simulink model "scheme1_analysis"  (R2019b)
settings: Solver=ode4  StartTime=0.0  StopTime=30  FixedStep=0.1  RelTol=1e-3
values from neighbouring files (symbols this model uses):
  Kd = K(3)    [solution.m]
  Ki = K(1)    [solution.m]
  Kp = K(2)    [solution.m]
settings Model: Creator=biannic  LastModifiedBy=biannic
settings DataIOCC: ReturnWorkspaceOutputs=off

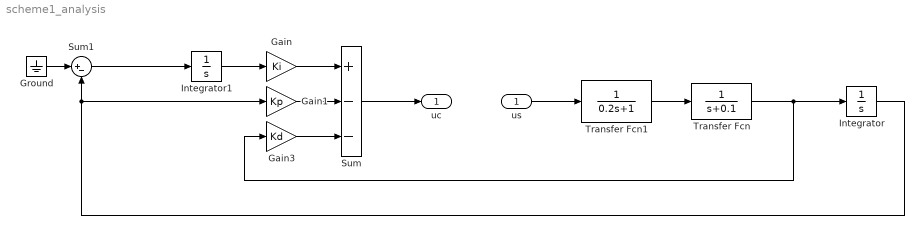
== system scheme1_analysis ==
  us : Inport
  Gain : Gain  Gain=Ki
  Gain1 : Gain  Gain=Kp
  Gain3 : Gain  Gain=Kd
  Ground : Ground
  Integrator : Integrator
  Integrator1 : Integrator
  Sum : Sum  Inputs=+--
  Sum1 : Sum  Inputs=|+-
  Transfer Fcn : TransferFcn  Denominator=[1 0.1]
  Transfer Fcn1 : TransferFcn  Denominator=[0.2 1]
  uc : Outport
  wires:
  Ground/1 -> Sum1/1
  Sum/1 -> uc/1
  us/1 -> Transfer Fcn1/1
  Transfer Fcn/1 -> Integrator/1, Gain3/1
  Integrator/1 -> Gain1/1, Sum1/2
  Sum1/1 -> Integrator1/1
  Transfer Fcn1/1 -> Transfer Fcn/1
  Gain3/1 -> Sum/3
  Gain1/1 -> Sum/2
  Gain/1 -> Sum/1
  Integrator1/1 -> Gain/1
